simulink model "yaw_damper_rev"  (R2013b)
settings: Solver=FixedStepDiscrete  SolverMode=SingleTasking  StartTime=0.0  StopTime=25  FixedStep=1/40  RelTol=1e-3
model workspace (MAT data in the model file):
  rateGain = Simulink.Parameter
  rateGain.Value = 2
  rateGain.DataType = 'auto'
  rateGain.Min = 0
  rateGain.Max = 1000
libraries: simulink x2
settings Model: CovSaveName=covdata_YawDamper  CovMetricSettings=dcmtrzoie  CovHTMLOptions=-sRT=1 -aTS=1 -bRG=1 -bTC=1 -hTR=1 -nFC=0 -scm=1 -bcm=1 -xEv=0  CovHtmlReporting=off  CovSaveSingleToWorkspaceVar=off  CovCumulativeVarName=covCumulativeData_YawDamper  CovCumulativeReport=on  CovReportOnPause=off  Creator=bpotter  LastModifiedBy=bpotter
settings DataIOCC: ExternalInput=rollIn  LimitDataPoints=off  SaveFormat=StructureWithTime  SaveOutput=off  DSMLogging=off  SaveTime=off  OutputSaveName=Ail_Cmd  SignalLoggingName=yaw_damper_logsout
settings OptimizationCC: BlockReduction=off  InlineParams=on  InlineInvariantSignals=on  EnhancedBackFolding=on  ExpressionDepthLimit=2147483647  EfficientFloat2IntCast=on  EfficientMapNaN2IntZero=off  OptimizeModelRefInitCode=on  MaxStackSize=inf
settings DebuggingCC: SignalInfNanChecking=error  SignalRangeChecking=error  ReadBeforeWriteMsg=EnableAllAsError  WriteAfterWriteMsg=EnableAllAsError  WriteAfterReadMsg=EnableAllAsError  AlgebraicLoopMsg=error  ArtificialAlgebraicLoopMsg=error  SaveWithDisabledLinksMsg=error  SaveWithParameterizedLinksMsg=error  UnderspecifiedInitializationDetection=Simplified  MergeDetectMultiDrivingBlocksExec=error  CheckExecutionContextPreStartOutputMsg=on  CheckExecutionContextRuntimeOutputMsg=on  BlockPriorityViolationMsg=error  MaxConsecutiveZCsMsg=warning  SolverPrmCheckMsg=error  InheritedTsInSrcMsg=error  DiscreteInheritContinuousMsg=error  SingleTaskRateTransMsg=error  TasksWithSamePriorityMsg=error  SigSpecEnsureSampleTimeMsg=error  CheckMatrixSingularityMsg=error  IntegerOverflowMsg=error  ParameterUnderflowMsg=error  ParameterPrecisionLossMsg=error  ParameterTunabilityLossMsg=error  UnderSpecifiedDataTypeMsg=error  UnnecessaryDatatypeConvMsg=warning  VectorMatrixConversionMsg=error  SignalLabelMismatchMsg=error  UnconnectedInputMsg=error  UnconnectedOutputMsg=error  UnconnectedLineMsg=error  SFcnCompatibilityMsg=error  UniqueDataStoreMsg=error  BusObjectLabelMismatch=error  RootOutportRequireBusObject=error  AssertControl=DisableAll  ModelReferenceIOMsg=error  ModelReferenceIOMismatchMessage=error  ModelReferenceCSMismatchMessage=warning  UnknownTsInhSupMsg=error  ModelReferenceDataLoggingMessage=error  ModelReferenceExtraNoncontSigs=none  StateNameClashWarn=warning  StrictBusMsg=ErrorOnBusTreatedAsVector  NonBusSignalsTreatedAsBus=error
settings HardwareCC: ProdIntDivRoundTo=Zero  ProdEndianess=BigEndian  ProdHWDeviceType=32-bit Embedded Processor  TargetHWDeviceType=32-bit Generic
settings RTWCC: SystemTargetFile=ert.tlc  TemplateMakefile=ert_default_tmf  Description=Embedded Coder  GenerateReport=on  RTWVerbose=off  ProcessScript=ert_make_rtw_hook  IncludeHyperlinkInReport=on  LaunchReport=on  PortableWordSizes=on  GenerateTraceInfo=on  GenerateTraceReport=on  GenerateTraceReportSl=on  GenerateTraceReportSf=on  GenerateTraceReportEml=on
settings CodeAppCC: ForceParamTrailComments=on  IgnoreCustomStorageClasses=off  MaxIdLength=63  MangleLength=4  CustomSymbolStrType=$N$R$M  InternalIdentifier=Classic  ReqsInCode=on
settings ERTTargetCC: CodeReplacementLibrary=ANSI_C  UtilityFuncGeneration=Shared location  IncludeMdlTerminateFcn=off  GeneratePreprocessorConditionals=Disable all  SuppressErrorStatus=on  SupportAbsoluteTime=off  SupportNonFinite=off  SupportComplex=off  ParenthesesLevel=Maximum  InlinedParameterPlacement=NonHierarchical  MultiInstanceErrorCode=None  ERTCustomFileTemplate=example_file_process.tlc  PreserveExpressionOrder=on  PreserveIfCondition=on

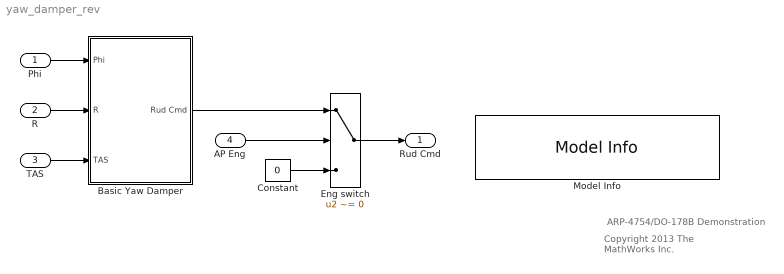
== system yaw_damper_rev ==
  note: Copyright 2013 The MathWorks Inc.
  note: ARP-4754/DO-178B Demonstration
  Phi : Inport  OutDataTypeStr=double  PortDimensions=1  SampleTime=1/40  Interpolate=off
  R : Inport  Port=2  OutDataTypeStr=double  PortDimensions=1  SampleTime=1/40  Interpolate=off
  TAS : Inport  Port=3  OutDataTypeStr=double  PortDimensions=1  SampleTime=1/40  Interpolate=off
  AP Eng : Inport  Port=4  OutDataTypeStr=boolean  PortDimensions=1  SampleTime=1/40  Interpolate=off
  Basic Yaw Damper : Subsystem  TreatAsAtomicUnit=on
      settings: RTWSystemCode=Inline
  Constant : Constant  Value=0  OutDataTypeStr=double
  Eng switch : Switch  Criteria=u2 ~= 0
  Model Info : simulink/Model-Wide Utilities/Model Info  InitialBlockCM=None  BlockCM=None  Frame=on  DisplayStringWithTags=|  HorizontalTextAlignment=Left  LeftAlignmentValue=0.02  SourceBlockDiagram=yaw_damper  TagMaxNumber=20
      | Yaw Damper
      | Author: %<LastModifiedBy>
      | Version: %<ModelVersion>
      | Date: %<LastModificationDate>
  Rud Cmd : Outport  OutDataTypeStr=double  PortDimensions=1  SampleTime=1/40
  wires:
  Phi/1 -> Basic Yaw Damper/1("Phi ")
  R/1 -> Basic Yaw Damper/2(R)
  Constant/1 -> Eng switch/3
  TAS/1 -> Basic Yaw Damper/3(TAS)
  Basic Yaw Damper/1(Rud Cmd) -> Eng switch/1
  AP Eng/1 -> Eng switch/2
  Eng switch/1 -> Rud Cmd/1

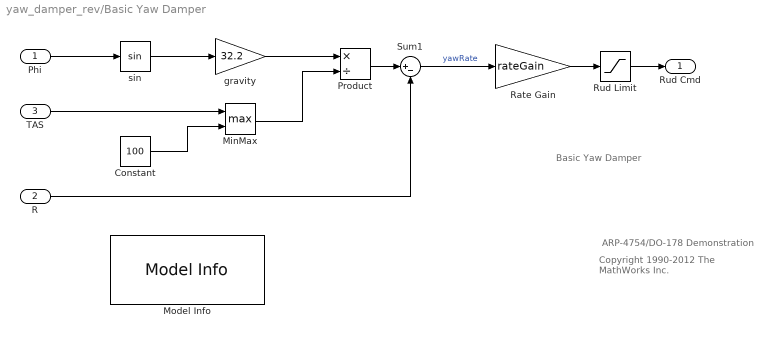
== system yaw_damper_rev/Basic Yaw Damper ==
  note: Basic Yaw Damper
  note: Copyright 1990-2012 The MathWorks Inc.
  note: ARP-4754/DO-178 Demonstration
  "Phi " : Inport
  R : Inport  Port=2
  TAS : Inport  Port=3
  Constant : Constant  Value=100
  MinMax : MinMax  Function=max  Inputs=2
  Model Info : simulink/Model-Wide Utilities/Model Info  InitialBlockCM=None  BlockCM=None  Frame=on  DisplayStringWithTags=|  HorizontalTextAlignment=Left  LeftAlignmentValue=0.02  SourceBlockDiagram=yaw_damper  TagMaxNumber=20
      | Yaw Damper
      | Author: %<LastModifiedBy>
      | Date: %<LastModificationDate>
      | Model Version: %<ModelVersion>
  Product : Product  Inputs=*/  RndMeth=Zero
  Rate Gain : Gain  Gain=rateGain
  Rud Limit : Saturate  UpperLimit=25  LowerLimit=-25
      settings: AttributesFormatString=%<LowerLimit> to %<UpperLimit> (deg)
  Sum1 : Sum  Inputs=|+-
  gravity : Gain  Gain=32.2
  sin : Trigonometry
  Rud Cmd : Outport
  wires:
  R/1 -> Sum1/2
  Sum1/1 -> Rate Gain/1  "yawRate"
  Rud Limit/1 -> Rud Cmd/1
  Rate Gain/1 -> Rud Limit/1
  "Phi "/1 -> sin/1
  sin/1 -> gravity/1
  Product/1 -> Sum1/1
  gravity/1 -> Product/1
  MinMax/1 -> Product/2
  TAS/1 -> MinMax/1
  Constant/1 -> MinMax/2
